simulink model "CARRR"  (R2025a)
settings: Solver=VariableStepAuto  StartTime=0.0  StopTime=1  RelTol=1e-3
values from neighbouring files (symbols this model uses):
  p1 = q0*Beta1    [OscCAR.m]
  p2 = q0*Beta2    [OscCAR.m]
  q0 = 1/(Beta1 + Beta2)    [OscCAR.m]
  q1 = q0*alpha1    [OscCAR.m]
  q2 = q0*alpha2    [OscCAR.m]
undefined symbols (not defined in the file or in its folder): dspblkCoreblockFVToolHelper, gcbh

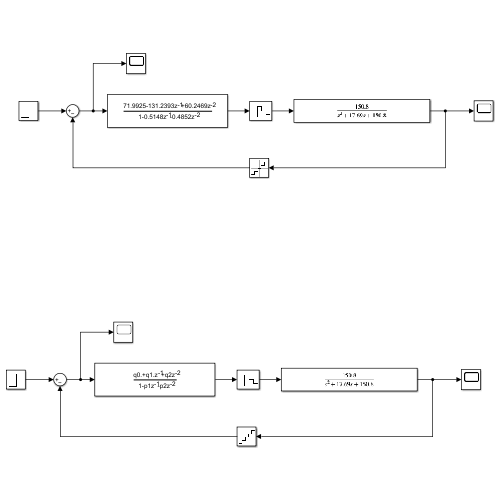
[thumbnail: Simulink's stored preview of the top-level diagram]
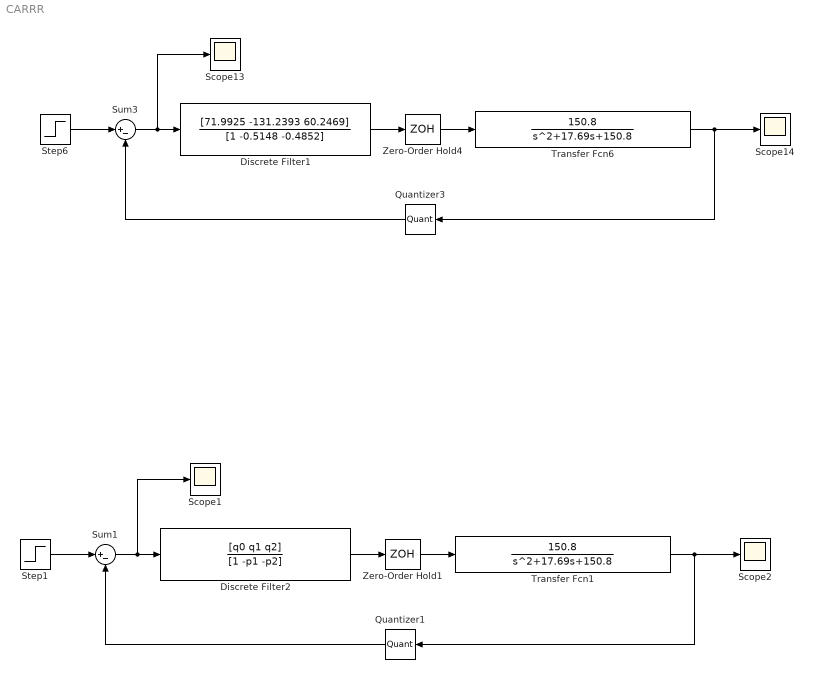
== system CARRR ==
  Discrete Filter1 : DiscreteFilter  LoadFcn=dspblkCoreblockFVToolHelper(gcbh,'load');  Numerator=[71.9925 -131.2393 60.2469]  Denominator=[1 -0.5148 -0.4852]
  Discrete Filter2 : DiscreteFilter  LoadFcn=dspblkCoreblockFVToolHelper(gcbh,'load');  Numerator=[q0 q1 q2]  Denominator=[1 -p1 -p2]
  Quantizer1 : Quantizer  QuantizationInterval=3.3/1024
  Quantizer3 : Quantizer  QuantizationInterval=3.3/1024
  Scope{1..2,13..14} (4 alike) : Scope
  Step1 : Step  Time=0  SampleTime=0
  Step6 : Step  Time=0  SampleTime=0
  Sum1 : Sum  Inputs=|+-
  Sum3 : Sum  Inputs=|+-
  Transfer Fcn1 : TransferFcn  Numerator=[150.8]  Denominator=[1 17.69 150.8]
  Transfer Fcn6 : TransferFcn  Numerator=[150.8]  Denominator=[1 17.69 150.8]
  Zero-Order Hold1 : ZeroOrderHold  SampleTime=0.01
  Zero-Order Hold4 : ZeroOrderHold  SampleTime=0.01
  wires:
  Sum3/1 -> Discrete Filter1/1, Scope13/1
  Transfer Fcn6/1 -> Quantizer3/1, Scope14/1
  Quantizer3/1 -> Sum3/2
  Discrete Filter1/1 -> Zero-Order Hold4/1
  Zero-Order Hold4/1 -> Transfer Fcn6/1
  Step6/1 -> Sum3/1
  Step1/1 -> Sum1/1
  Zero-Order Hold1/1 -> Transfer Fcn1/1
  Discrete Filter2/1 -> Zero-Order Hold1/1
  Quantizer1/1 -> Sum1/2
  Transfer Fcn1/1 -> Scope2/1, Quantizer1/1
  Sum1/1 -> Scope1/1, Discrete Filter2/1
